simulink model "System"  (R2021a)
settings: Solver=VariableStepAuto  StartTime=0  StopTime=60*60*50  RelTol=1e-2
undefined symbols (not defined in the file): b_g, C_g, C_m_int, c_w, COPMAX, COPMIN, delta, delta_t, DTemp, hmint, K, KTC, mMAX, PelMAX, S_g, Smint, Tgeo, Toutmax
libraries: pid_lib x1
settings Model: PauseTimes=0  Creator=Fabrizio  LastModifiedBy=Fabrizio
settings DataIOCC: SaveFormat=StructureWithTime
settings OptimizationCC: BlockReduction=off  BufferReuse=off
settings DebuggingCC: AlgebraicLoopMsg=none  UnconnectedInputMsg=none  UnconnectedOutputMsg=none  UnconnectedLineMsg=none  SFMachineParentedDataDiag=warning

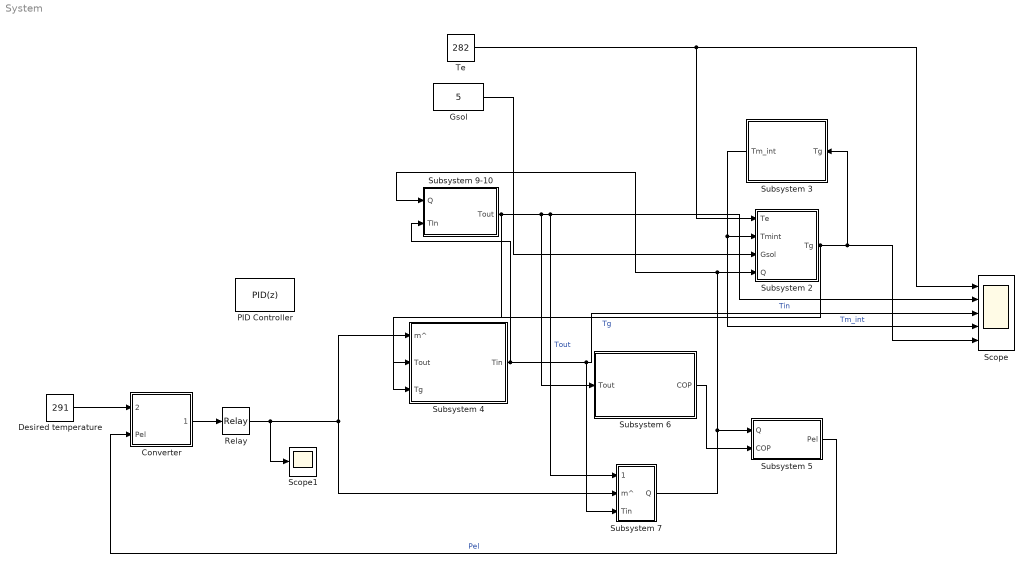
== system System ==
  Converter : Subsystem
      settings: PortSchema="{\"entries\":[{\"content\":{\"sides\":[{\"content\":{\"connectorIds\":[]},\"type\":\"ConnectorPlacement.EquallySpacedRectSide\",\"uuid\":\"f0b54d86-226c-4f72-9e43-8ae001c7af10\"},{\"content\":{\"connectorIds\":[],\"side\":\"RIGHT\"},\"type\":\"ConnectorPlacement.EquallySpacedRectSide\",\"uuid\":\"cee7571e-abcc-434e-9af0-036ec0a70a3b\"},{\"content\":{\"connectorIds\":[\"In1\",\"In2\"],\"side\":\"TOP\"},\"type\":\"ConnectorPlacement.EquallySpacedRectSide\",\"uuid\":\"0ebf61e3-8416-4076-8685-d65d90996bf2\"},{\"content\":{\"connectorIds\":[\"Out1\"],\"side\":\"BOTTOM\"},\"type\":\"ConnectorPlacement.EquallySpacedRectSide\",\"uuid\":\"95dc95ec-af1a-499b-8498-c37cf51ba5fb\"}]},\"type\":\"ConnectorPlacement.EquallySpacedConnector\",\"uuid\":\"2168eb8c-c2af-4bd4-b50f-a389009ab49a\"}],\"packageUris\":[\"http://schema.mathworks.com/mf0/Connector/R2020b\"],\"version\":\"1.0\"}"
  Desired temperature : Constant  Value=291
  Gsol : Constant  Value=5
  PID Controller : pid_lib/PID Controller  Controller=PID  Form=Parallel  TimeDomain=Discrete-time  UseExternalTs=off  SampleTime=delta_t  IntegratorMethod=Forward Euler  FilterMethod=Forward Euler  ControllerParametersSource=internal  P=-711399070870829  I=-7904434120786.99  D=0  UseFilter=on  N=100  TunerSelectOption=Transfer Function Based (PID Tuner App)  InitialConditionSource=internal  InitialConditionForIntegrator=0  InitialConditionForFilter=0  DifferentiatorICPrevScaledInput=0  ExternalReset=none  TrackingMode=off  Kt=1  LimitOutput=on  SatLimitsSource=internal  UpperSaturationLimit=mMAX  LowerSaturationLimit=1  LinearizeAsGain=on  AntiWindupMode=none  Kb=1  POutMin=[]  POutMax=[]  IOutMin=[]  IOutMax=[]  DOutMin=[]  DOutMax=[]  NOutMin=[]  NOutMax=[]  SumOutMin=[]  SumOutMax=[]  SaturationOutMin=[]  SaturationOutMax=[]  PParamMin=[]  PParamMax=[]  IParamMin=[]  IParamMax=[]  DParamMin=[]  DParamMax=[]  NParamMin=[]  NParamMax=[]  KbParamMin=[]  KbParamMax=[]  KtParamMin=[]  KtParamMax=[]  KbOutMin=[]  KbOutMax=[]  KtOutMin=[]  KtOutMax=[]  IntegratorOutMin=[]  IntegratorOutMax=[]  FilterOutMin=[]  FilterOutMax=[]  SumI1OutMin=[]  SumI1OutMax=[]  SumI2OutMin=[]  SumI2OutMax=[]  SumI3OutMin=[]  SumI3OutMax=[]  SumI4OutMin=[]  SumI4OutMax=[]  SumDOutMin=[]  SumDOutMax=[]  DifferentiatorOutMin=[]  DifferentiatorOutMax=[]  FilterDiffOutCoefMin=[]  FilterDiffOutCoefMax=[]  ReciprocalOutMin=[]  ReciprocalOutMax=[]  SumDenOutMin=[]  SumDenOutMax=[]  SumNumOutMin=[]  SumNumOutMax=[]  DivideOutMin=[]  DivideOutMax=[]  UdiffTsProdOutMin=[]  UdiffTsProdOutMax=[]  NTsProdOutMin=[]  NTsProdOutMax=[]  UintegralTsProdOutMin=[]  UintegralTsProdOutMax=[]  UngainTsProdOutMin=[]  UngainTsProdOutMax=[]  IntegratorContinuousStateAttributes=''  IntegratorStateMustResolveToSignalObject=off  IntegratorRTWStateStorageClass=Auto  FilterContinuousStateAttributes=''  FilterStateMustResolveToSignalObject=off  FilterRTWStateStorageClass=Auto  ParallelPVariant=InternalParameters  IdealPVariant=Disabled  IVariant=InternalParameters  DVariant=InternalParameters  IntegratorVariant=Discrete  SatVariant=Enabled  AWVariant=Passthrough  PCopyVariant=Disabled  TRVariant=Disabled  FdbkBlocksVariant=Forward  IdealPFdbkVariant=Disabled  SatFdbkVariant=Disabled  DerivativeFilterVariant=ForwardEulerFilter  NVariant=InternalParameters  NCopyVariant=Disabled  FilterICVariant=InternalICsFilter  IntegratorICVariant=InternalICs  ExternalResetVariant=Disabled  TRSumVariant=Passthrough  SumFdbkVariant=Disabled  SumVariant=Sum_PID  TsampFilterVariant=InternalTs  TsampNgainVariant=Passthrough  TsampIntegralVariant=Passthrough  ExternalSaturationOutDataTypeStr=Inherit: Same as second input
  Relay : Relay  OnSwitchValue=1  OffSwitchValue=0  OnOutputValue=mMAX*10
  Scope : Scope  NumInputPorts=5
  Scope1 : Scope
  Subsystem 2 : Subsystem
  Subsystem 3 : Subsystem
  Subsystem 4 : Subsystem
  Subsystem 5 : Subsystem
  Subsystem 6 : Subsystem
  Subsystem 7 : Subsystem
  Subsystem 9-10 : Subsystem
  Te : Constant  Value=282
  wires:
  Te/1 -> Scope/1, Subsystem 2/1(Te)
  Gsol/1 -> Subsystem 2/3(Gsol)
  Subsystem 3/1(Tm_int) -> Scope/4, Subsystem 2/2(Tmint)  "Tm_int"
  Subsystem 6/1(COP) -> Subsystem 5/2(COP)
  Relay/1 -> Subsystem 4/1(m^), Subsystem 7/2(m^), Scope1/1
  Subsystem 7/1(Q) -> Subsystem 5/1(Q), Subsystem 9-10/1(Q), Subsystem 2/4(Q)
  Converter/1(delta_m^) -> Relay/1
  Desired temperature/1 -> Converter/2(rif Temp)
  Subsystem 5/1(Pel) -> Converter/1(Pel)  "Pel"
  Subsystem 2/1(Tg) -> Subsystem 3/1(Tg), Scope/5, Subsystem 4/3(Tg)  "Tg"
  Subsystem 4/1(Tin) -> Subsystem 7/3(Tin), Scope/3, Subsystem 9-10/2(TIn)  "Tin"
  Subsystem 9-10/1(Tout) -> Scope/2, Subsystem 7/1(Tout), Subsystem 6/1(Tout), Subsystem 4/2(Tout)  "Tout"

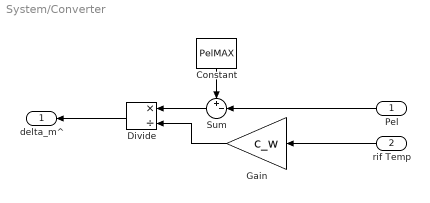
== system System/Converter ==
  Pel : Inport
  rif Temp : Inport  Port=2
  Constant : Constant  Value=PelMAX
  Divide : Product  Inputs=*/
  Gain : Gain  Gain=c_w
  Sum : Sum  Inputs=+-|
  delta_m^ : Outport
  wires:
  Gain/1 -> Divide/2
  rif Temp/1 -> Gain/1
  Divide/1 -> delta_m^/1
  Sum/1 -> Divide/1
  Pel/1 -> Sum/2
  Constant/1 -> Sum/1

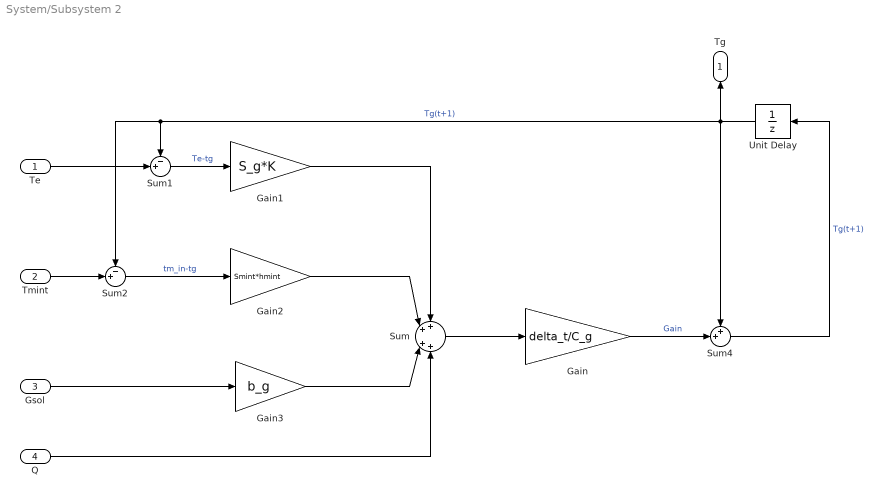
== system System/Subsystem 2 ==
  Te : Inport
  Tmint : Inport  Port=2
  Gsol : Inport  Port=3
  Q : Inport  Port=4
  Gain : Gain  Gain=delta_t/C_g
  Gain1 : Gain  Gain=S_g*K
  Gain2 : Gain  Gain=Smint*hmint
  Gain3 : Gain  Gain=b_g
  Sum : Sum  Inputs=++|++
  Sum1 : Sum  Inputs=-+|
  Sum2 : Sum  Inputs=-+|
  Sum4 : Sum  Inputs=++|
  Unit Delay : UnitDelay  InitialCondition=288  SampleTime=delta_t  HasFrameUpgradeWarning=on
  Tg : Outport
  wires:
  Sum2/1 -> Gain2/1  "tm_in-tg"
  Sum/1 -> Gain/1
  Gain1/1 -> Sum/1
  Gain2/1 -> Sum/2
  Gain3/1 -> Sum/3
  Sum1/1 -> Gain1/1  "Te-tg"
  Sum4/1 -> Unit Delay/1  "Tg(t+1)"
  Te/1 -> Sum1/2
  Gain/1 -> Sum4/2  "Gain"
  Tmint/1 -> Sum2/2
  Gsol/1 -> Gain3/1
  Q/1 -> Sum/4
  Unit Delay/1 -> Tg/1, Sum2/1, Sum1/1, Sum4/1  "Tg(t+1)"

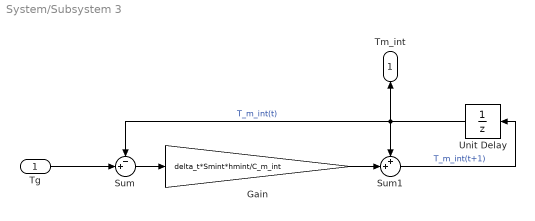
== system System/Subsystem 3 ==
  Tg : Inport
  Gain : Gain  Gain=delta_t*Smint*hmint/C_m_int
  Sum : Sum  Inputs=-+|
  Sum1 : Sum  Inputs=++|
  Unit Delay : UnitDelay  InitialCondition=273+15  SampleTime=delta_t  HasFrameUpgradeWarning=on
  Tm_int : Outport
  wires:
  Tg/1 -> Sum/2
  Sum/1 -> Gain/1
  Gain/1 -> Sum1/2
  Sum1/1 -> Unit Delay/1  "T_m_int(t+1)"
  Unit Delay/1 -> Tm_int/1, Sum1/1, Sum/1  "T_m_int(t)"

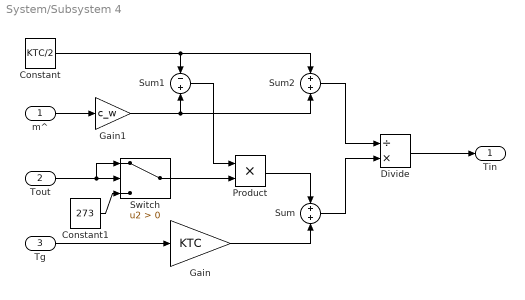
== system System/Subsystem 4 ==
  m^ : Inport
  Tout : Inport  Port=2
  Tg : Inport  Port=3
  Constant : Constant  Value=KTC/2
  Constant1 : Constant  Value=273
  Divide : Product  Inputs=/*
  Gain : Gain  Gain=KTC
  Gain1 : Gain  Gain=c_w
  Product : Product
  Sum : Sum  Inputs=+|+
  Sum1 : Sum  Inputs=-|+
  Sum2 : Sum  Inputs=+|+
  Switch : Switch  Criteria=u2 > Threshold
  Tin : Outport
  wires:
  Tg/1 -> Gain/1
  Gain/1 -> Sum/2
  m^/1 -> Gain1/1
  Constant/1 -> Sum2/1, Sum1/1
  Tout/1 -> Switch/1, Switch/2
  Sum1/1 -> Product/1
  Product/1 -> Sum/1
  Divide/1 -> Tin/1
  Sum/1 -> Divide/2
  Gain1/1 -> Sum2/2, Sum1/2
  Sum2/1 -> Divide/1
  Constant1/1 -> Switch/3
  Switch/1 -> Product/2

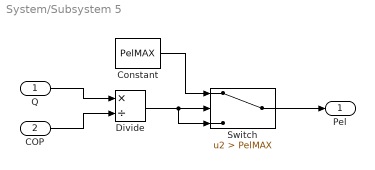
== system System/Subsystem 5 ==
  Q : Inport
  COP : Inport  Port=2
  Constant : Constant  Value=PelMAX
  Divide : Product  Inputs=*/
  Switch : Switch  Criteria=u2 > Threshold  Threshold=PelMAX
  Pel : Outport
  wires:
  Divide/1 -> Switch/3, Switch/2
  COP/1 -> Divide/2
  Q/1 -> Divide/1
  Switch/1 -> Pel/1
  Constant/1 -> Switch/1

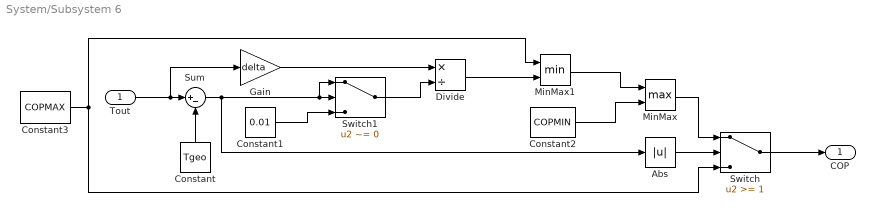
== system System/Subsystem 6 ==
  Tout : Inport
  Abs : Abs
  Constant : Constant  Value=Tgeo
  Constant1 : Constant  Value=0.01
  Constant2 : Constant  Value=COPMIN
  Constant3 : Constant  Value=COPMAX
  Divide : Product  Inputs=*/
  Gain : Gain  Gain=delta
  MinMax : MinMax  Function=max  Inputs=2
  MinMax1 : MinMax  Inputs=2
  Sum : Sum  Inputs=|+-
  Switch : Switch  Threshold=1
  Switch1 : Switch  Criteria=u2 ~= 0
  COP : Outport
  wires:
  Switch/1 -> COP/1
  Abs/1 -> Switch/2
  Sum/1 -> Switch1/1, Switch1/2, Abs/1
  Constant/1 -> Sum/2
  Constant3/1 -> Switch/3, MinMax1/1
  Tout/1 -> Gain/1, Sum/1
  MinMax/1 -> Switch/1
  Constant2/1 -> MinMax/2
  MinMax1/1 -> MinMax/1
  Divide/1 -> MinMax1/2
  Gain/1 -> Divide/1
  Switch1/1 -> Divide/2
  Constant1/1 -> Switch1/3

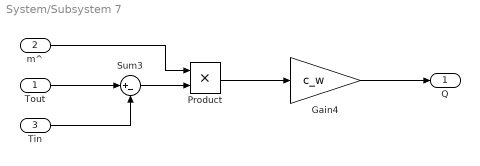
== system System/Subsystem 7 ==
  Tout : Inport
  m^ : Inport  Port=2
  Tin : Inport  Port=3
  Gain4 : Gain  Gain=c_w
  Product : Product
  Sum3 : Sum  Inputs=|+-
  Q : Outport
  wires:
  Product/1 -> Gain4/1
  Sum3/1 -> Product/2
  Tout/1 -> Sum3/1
  Gain4/1 -> Q/1
  m^/1 -> Product/1
  Tin/1 -> Sum3/2

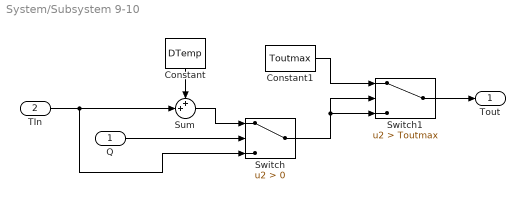
== system System/Subsystem 9-10 ==
  Q : Inport
  TIn : Inport  Port=2
  Constant : Constant  Value=DTemp
  Constant1 : Constant  Value=Toutmax
  Sum : Sum  Inputs=++|
  Switch : Switch  Criteria=u2 > Threshold
  Switch1 : Switch  Criteria=u2 > Threshold  Threshold=Toutmax
  Tout : Outport
  wires:
  Q/1 -> Switch/2
  Sum/1 -> Switch/1
  TIn/1 -> Switch/3, Sum/2
  Constant/1 -> Sum/1
  Switch1/1 -> Tout/1
  Switch/1 -> Switch1/3, Switch1/2
  Constant1/1 -> Switch1/1
